simulink library "communications_lib"  (Simulink 8.1)
settings: Solver=ode45  StartTime=0.0  StopTime=10.0  RelTol=1e-3
values from neighbouring files (symbols this model uses):
  Ts = 100E-6    (= 0.0001)    [BANSHEE_init.m]    (also in Ghost_init.m)
libraries: goose_lib x6, rtlab x4, power_quality_lib x4, rtio_generic_modbus x2, DMS_slave_lib x2, LoadProfiles_lib x2, NREL_UDP_lib x2
(part 2 of 2)

== system communications_lib/SS_COMMUNICATION_34_NoGoose/MGC_controller/Subsystem ==
  Bus Selector18 : BusSelector  OutputSignals=F3_CB_CTRL
  Bus Selector19 : BusSelector  OutputSignals=signal11
  Constant : Constant  Value=0
  Constant1 : Constant  Value=0
  Mux : Mux  Inputs=3
  Out1 : Outport
  wires:
  Constant1/1 -> Mux/2
  Constant/1 -> Mux/1
  [F3_RELAY_OUT] -> Bus Selector18/1
  Mux/1 -> Out1/1
  Bus Selector18/1 -> Bus Selector19/1  "<F3_CB_CTRL>"
  Bus Selector19/1 -> Mux/3  "<signal11>"

== system communications_lib/SS_COMMUNICATION_34_NoGoose/Misc_data/Subsystem ==
  In1 : Inport
  Bus Selector28 : BusSelector  OutputSignals=F3.LOAD_DATA.F3_I6.kw,F4.LOAD_DATA.F4_I7.kw,F4.LOAD_DATA.F4_I8.kw,F3.LOAD_DATA.F3_P4.kw,F3.LOAD_DATA.F3_P6.kw,F4.LOAD_DATA.F4_P7.kw,F4.LOAD_DATA.F4_P8.kw,F3.LOAD_DATA.F3_C5.kw,F3.LOAD_DATA.F3_C6.kw,F4.LOAD_DATA.F4_C7.kw,F4.LOAD_DATA.F4_C8.kw,F4.LOAD_DATA.F4_C9.kw
  Constant : Constant  Value=0
  Mux : Mux  Inputs=25
  Out1 : Outport
  wires:
  Constant/1 -> Mux/1, Mux/2, Mux/9, Mux/18, Mux/20, Mux/19, Mux/17, Mux/13, Mux/11, Mux/10, Mux/5, Mux/4, Mux/3
  Mux/1 -> Out1/1
  Bus Selector28/5 -> Mux/14  "<kw>"
  Bus Selector28/6 -> Mux/15  "<kw>"
  Bus Selector28/3 -> Mux/8  "<kw>"
  Bus Selector28/1 -> Mux/6  "<kw>"
  Bus Selector28/7 -> Mux/16  "<kw>"
  Bus Selector28/12 -> Mux/25  "<kw>"
  Bus Selector28/10 -> Mux/23  "<kw>"
  Bus Selector28/11 -> Mux/24  "<kw>"
  Bus Selector28/9 -> Mux/22  "<kw>"
  Bus Selector28/2 -> Mux/7  "<kw>"
  Bus Selector28/8 -> Mux/21  "<kw>"
  Bus Selector28/4 -> Mux/12  "<kw>"
  In1/1 -> Bus Selector28/1

== system communications_lib/SS_COMMUNICATION_34_NoGoose/Misc_data/Subsystem1 ==
  In1 : Inport
  Bus Selector29 : BusSelector  OutputSignals=F3.LOAD_DATA.F3_I6.VRMSLL,F4.LOAD_DATA.F4_I7.VRMSLL,F4.LOAD_DATA.F4_I8.VRMSLL,F3.LOAD_DATA.F3_P4.VRMSLL,F3.LOAD_DATA.F3_P6.VRMSLL,F4.LOAD_DATA.F4_P7.VRMSLL,F4.LOAD_DATA.F4_P8.VRMSLL,F3.LOAD_DATA.F3_C5.VRMSLL,F3.LOAD_DATA.F3_C6.VRMSLL,F4.LOAD_DATA.F4_C7.VRMSLL,F4.LOAD_DATA.F4_C8.VRMSLL,F4.LOAD_DATA.F4_C9.VRMSLL
  Constant : Constant  Value=0
  Mux : Mux  Inputs=25
  Out1 : Outport
  wires:
  Constant/1 -> Mux/17, Mux/18, Mux/20, Mux/19, Mux/13, Mux/11, Mux/10, Mux/9, Mux/5, Mux/4, Mux/3, Mux/2, Mux/1
  Bus Selector29/5 -> Mux/14  "<VRMSLL>"
  Bus Selector29/6 -> Mux/15  "<VRMSLL>"
  Bus Selector29/7 -> Mux/16  "<VRMSLL>"
  Bus Selector29/8 -> Mux/21  "<VRMSLL>"
  Bus Selector29/9 -> Mux/22  "<VRMSLL>"
  Bus Selector29/10 -> Mux/23  "<VRMSLL>"
  Bus Selector29/11 -> Mux/24  "<VRMSLL>"
  Bus Selector29/12 -> Mux/25  "<VRMSLL>"
  Bus Selector29/1 -> Mux/6  "<VRMSLL>"
  Bus Selector29/3 -> Mux/8  "<VRMSLL>"
  Bus Selector29/2 -> Mux/7  "<VRMSLL>"
  Bus Selector29/4 -> Mux/12  "<VRMSLL>"
  In1/1 -> Bus Selector29/1
  Mux/1 -> Out1/1

== system communications_lib/SS_COMMUNICATION_34_NoGoose/Relay_data/ExtractF3 ==
  In1 : Inport
  Bus Selector47 : BusSelector  OutputSignals=F3_CB_1,F3_CB_2,F3_CB_3,F3_CB_4,F3_CB_5,F3_CB_6,F3_CB_7,F3_CB_8,F3_CB_9,F3_CB_10
  Bus Selector{48..53,56,58..59,61} (10 alike) : BusSelector  OutputSignals=m.kw,m.kvar,m.Vpu,m.Hz,m.status  OutputAsBus=on
  Mux13 : Mux  Inputs=10
  Out1 : Outport
  wires:
  Bus Selector61/1 -> Mux13/3
  Bus Selector59/1 -> Mux13/10
  Bus Selector47/5 -> Bus Selector51/1  "<F3_CB_5>"
  Bus Selector47/10 -> Bus Selector59/1  "<F3_CB_10>"
  Bus Selector49/1 -> Mux13/2
  Bus Selector47/2 -> Bus Selector49/1  "<F3_CB_2>"
  Bus Selector47/3 -> Bus Selector61/1  "<F3_CB_3>"
  Bus Selector47/9 -> Bus Selector58/1  "<F3_CB_9>"
  Bus Selector47/8 -> Bus Selector56/1  "<F3_CB_8>"
  Bus Selector47/7 -> Bus Selector53/1  "<F3_CB_7>"
  Bus Selector47/6 -> Bus Selector52/1  "<F3_CB_6>"
  Bus Selector58/1 -> Mux13/9
  Bus Selector56/1 -> Mux13/8
  Bus Selector52/1 -> Mux13/6
  Mux13/1 -> Out1/1
  In1/1 -> Bus Selector47/1
  Bus Selector50/1 -> Mux13/4
  Bus Selector47/1 -> Bus Selector48/1  "<F3_CB_1>"
  Bus Selector47/4 -> Bus Selector50/1  "<F3_CB_4>"
  Bus Selector53/1 -> Mux13/7
  Bus Selector48/1 -> Mux13/1
  Bus Selector51/1 -> Mux13/5

== system communications_lib/SS_COMMUNICATION_34_NoGoose/Relay_data/ExtractF4 ==
  In1 : Inport
  Bus Selector47 : BusSelector  OutputSignals=F4_CB_1,F4_CB_2,F4_CB_3,F4_CB_4,F4_CB_5,F4_CB_6
  Bus Selector{48..52,61} (6 alike) : BusSelector  OutputSignals=m.kw,m.kvar,m.Vpu,m.Hz,m.status  OutputAsBus=on
  Mux13 : Mux  Inputs=6
  Out1 : Outport
  wires:
  Bus Selector51/1 -> Mux13/5
  Bus Selector48/1 -> Mux13/1
  Bus Selector47/4 -> Bus Selector50/1  "<F4_CB_4>"
  Bus Selector47/1 -> Bus Selector48/1  "<F4_CB_1>"
  Bus Selector50/1 -> Mux13/4
  In1/1 -> Bus Selector47/1
  Mux13/1 -> Out1/1
  Bus Selector52/1 -> Mux13/6
  Bus Selector47/6 -> Bus Selector52/1  "<F4_CB_6>"
  Bus Selector47/3 -> Bus Selector61/1  "<F4_CB_3>"
  Bus Selector47/2 -> Bus Selector49/1  "<F4_CB_2>"
  Bus Selector49/1 -> Mux13/2
  Bus Selector47/5 -> Bus Selector51/1  "<F4_CB_5>"
  Bus Selector61/1 -> Mux13/3

== system communications_lib/SS_COMMUNICATION_34_NoGoose/Relay_data/Subsystem ==
  F3 : Inport
  Bus Selector3 : BusSelector  OutputSignals=F3_PCC
  Bus Selector4 : BusSelector  OutputSignals=m.kw,m.kvar,m.Vpu,m.Hz,m.status  OutputAsBus=on
  Constant1 : Constant  Value=zeros(1,5)
  Constant3 : Constant  Value=zeros(1,5)
  Mux : Mux  Inputs=3
  Out1 : Outport
  wires:
  Constant1/1 -> Mux/2
  Mux/1 -> Out1/1
  Bus Selector4/1 -> Mux/3
  F3/1 -> Bus Selector3/1
  Bus Selector3/1 -> Bus Selector4/1  "<F3_PCC>"
  Constant3/1 -> Mux/1

== system communications_lib/SS_COMMUNICATION_34_NoGoose/Relay_data/Subsystem1 ==
  F3 : Inport
  F4 : Inport  Port=2
  Bus Selector10 : BusSelector  OutputSignals=m.kw,m.kvar,m.Vpu,m.Hz,m.status  OutputAsBus=on
  Bus Selector11 : BusSelector  OutputSignals=cb.relay_out
  Bus Selector12 : BusSelector  OutputSignals=CB_meas.relay_out.m.kw,CB_meas.relay_out.m.kvar,CB_meas.relay_out.m.Vpu,CB_meas.relay_out.m.Hz,CB_meas.cb_meas.Status  OutputAsBus=on
  Bus Selector16 : BusSelector  OutputSignals=cb.relay_out
  Bus Selector17 : BusSelector  OutputSignals=CB_meas.relay_out.m.kw,CB_meas.relay_out.m.kvar,CB_meas.relay_out.m.Vpu,CB_meas.relay_out.m.Hz,CB_meas.cb_meas.Status  OutputAsBus=on
  Bus Selector3 : BusSelector  OutputSignals=NG_CHP_DATA
  Bus Selector4 : BusSelector  OutputSignals=m.kw,m.kvar,m.Vpu,m.Hz,m.status  OutputAsBus=on
  Bus Selector9 : BusSelector  OutputSignals=GEN3_DATA,ESS_DATA,PV_DATA
  Constant1 : Constant  Value=zeros(1,5)
  Constant2 : Constant  Value=zeros(1,5)
  Constant3 : Constant  Value=zeros(1,5)
  Mux : Mux  Inputs=7
  Out1 : Outport
  wires:
  Constant2/1 -> Mux/3
  Constant1/1 -> Mux/2
  Bus Selector9/2 -> Bus Selector17/1  "<ESS_DATA>"
  Bus Selector16/1 -> Bus Selector4/1  "<relay_out>"
  Bus Selector12/1 -> Mux/7
  Bus Selector9/3 -> Bus Selector12/1  "<PV_DATA>"
  Bus Selector17/1 -> Mux/6
  Bus Selector10/1 -> Mux/5
  Bus Selector11/1 -> Bus Selector10/1  "<relay_out>"
  Bus Selector9/1 -> Bus Selector11/1  "<GEN3_DATA>"
  F4/1 -> Bus Selector9/1
  Constant3/1 -> Mux/1
  Bus Selector3/1 -> Bus Selector16/1  "<NG_CHP_DATA>"
  F3/1 -> Bus Selector3/1
  Bus Selector4/1 -> Mux/4
  Mux/1 -> Out1/1
